simulink model "Duocopter_APID_Model"  (R2024b)
settings: Solver=VariableStepAuto  StartTime=0.0  StopTime=10.0  RelTol=1e-3
undefined symbols (not defined in the file): DiscIntNeverNeededParam, Discrete, Time
libraries: ctrlSharedLib x1, slpidlib x1
settings Model: Creator=charlemagne  LastModifiedBy=Nicol

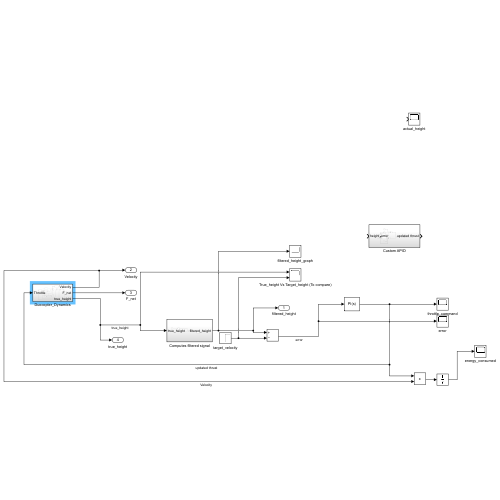
[thumbnail: Simulink's stored preview of the top-level diagram]
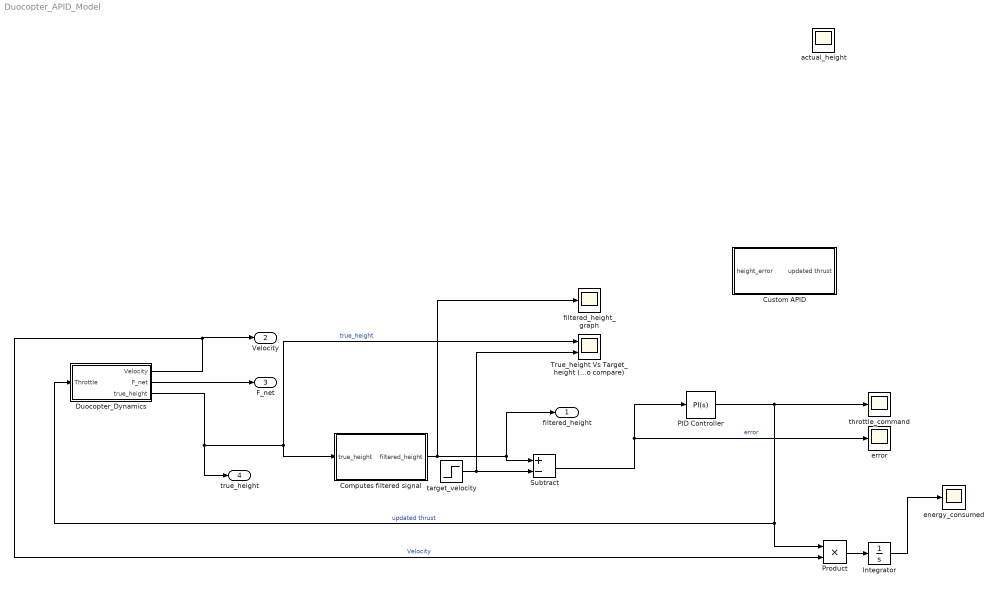
== system Duocopter_APID_Model ==
  Computes filtered signal : Subsystem
  Custom APID : Subsystem
  Duocopter_Dynamics : Subsystem
  Integrator : Integrator
  PID Controller : slpidlib/PID Controller  Controller=PI  Form=Parallel  TimeDomain=Continuous-time  UseExternalTs=off  SampleTime=-1  IntegratorMethod=Forward Euler  FilterMethod=Forward Euler  ControllerParametersSource=internal  P=120  I=80  UseKiTs=off  D=0  UseExternalDerivativeSource=off  N=100  UseFilter=on  TunerSelectOption=Transfer Function Based (PID Tuner App)  InitialConditionSource=internal  InitialConditionForIntegrator=0  InitialConditionForFilter=0  DifferentiatorICPrevScaledInput=0  ExternalReset=none  TrackingMode=off  Kt=1  LimitOutput=off  SatLimitsSource=internal  UpperSaturationLimit=inf  LowerSaturationLimit=-inf  LinearizeAsGain=on  AntiWindupMode=none  Kb=1  LimitIntegrator=off  UpperIntegratorSaturationLimit=inf  LowerIntegratorSaturationLimit=-inf  POutMin=[]  POutMax=[]  IOutMin=[]  IOutMax=[]  DOutMin=[]  DOutMax=[]  NOutMin=[]  NOutMax=[]  SumOutMin=[]  SumOutMax=[]  SaturationOutMin=[]  SaturationOutMax=[]  PParamMin=[]  PParamMax=[]  IParamMin=[]  IParamMax=[]  DParamMin=[]  DParamMax=[]  NParamMin=[]  NParamMax=[]  KbParamMin=[]  KbParamMax=[]  KtParamMin=[]  KtParamMax=[]  KbOutMin=[]  KbOutMax=[]  KtOutMin=[]  KtOutMax=[]  IntegratorOutMin=[]  IntegratorOutMax=[]  FilterOutMin=[]  FilterOutMax=[]  SumI1OutMin=[]  SumI1OutMax=[]  SumI2OutMin=[]  SumI2OutMax=[]  SumI3OutMin=[]  SumI3OutMax=[]  SumI4OutMin=[]  SumI4OutMax=[]  SumDOutMin=[]  SumDOutMax=[]  DifferentiatorOutMin=[]  DifferentiatorOutMax=[]  FilterDiffOutCoefMin=[]  FilterDiffOutCoefMax=[]  ReciprocalOutMin=[]  ReciprocalOutMax=[]  SumDenOutMin=[]  SumDenOutMax=[]  SumNumOutMin=[]  SumNumOutMax=[]  DivideOutMin=[]  DivideOutMax=[]  UdiffTsProdOutMin=[]  UdiffTsProdOutMax=[]  NTsProdOutMin=[]  NTsProdOutMax=[]  UintegralTsProdOutMin=[]  UintegralTsProdOutMax=[]  UngainTsProdOutMin=[]  UngainTsProdOutMax=[]  ClampingZeroOutDataTypeStr=Inherit: Inherit via back propagation  ClampingZeroOutMin=[]  ClampingZeroOutMax=[]  FilterDenConstantOutDataTypeStr=Inherit: Inherit via back propagation  FilterDenConstantOutMin=[]  FilterDenConstantOutMax=[]  PCopyOutDataTypeStr=Inherit: Inherit via back propagation  PCopyOutMin=[]  PCopyOutMax=[]  NCopyOutDataTypeStr=Inherit: Inherit via back propagation  NCopyOutMin=[]  NCopyOutMax=[]  IntegratorContinuousStateAttributes=''  IntegratorStateMustResolveToSignalObject=off  IntegratorRTWStateStorageClass=Auto  FilterContinuousStateAttributes=''  FilterStateMustResolveToSignalObject=off  FilterRTWStateStorageClass=Auto  ParallelPVariant=InternalParameters  IdealPVariant=Disabled  IVariant=InternalParameters  DVariant=Disabled  IntegratorVariant=Continuous  SatVariant=Disabled  AWVariant=Passthrough  PCopyVariant=Disabled  TRVariant=Disabled  FdbkBlocksVariant=Forward  IdealPFdbkVariant=Disabled  SatFdbkVariant=Disabled  DerivativeFilterVariant=Disabled  NVariant=Disabled  NCopyVariant=Disabled_SignalSpec  FilterICVariant=Disabled  IntegratorICVariant=InternalICs  ExternalResetVariant=Disabled  TRSumVariant=Passthrough  SumFdbkVariant=Disabled  SumVariant=Sum_PI  TsampFilterVariant=InternalTs  TsampNgainVariant=Passthrough  TsampIntegralVariant=Disabled_SignalSpec  ExternalSaturationOutDataTypeStr=Inherit: Same as second input  DerivativeSourceVariant=Disabled  PreIntVariant=InternalPreInt
  Product : Product
  Subtract : Sum  Inputs=+-
  True_height Vs Target_height (To compare) : Scope  NumInputPorts=2
  actual_height : Scope
  energy_consumed : Scope
  error : Scope
  filtered_height_graph : Scope
  target_velocity : Step  SampleTime=0
  throttle_command : Scope
  filtered_height : Outport
  Velocity : Outport  Port=2
  F_net : Outport  Port=3
  true_height : Outport  Port=4
  wires:
  Computes filtered signal/1(filtered_height) -> filtered_height_graph/1, filtered_height/1, Subtract/1
  Duocopter_Dynamics/1(Velocity) -> Product/2, Velocity/1  "Velocity"
  Duocopter_Dynamics/2(F_net) -> F_net/1
  Duocopter_Dynamics/3(true_height) -> true_height/1, True_height Vs Target_height (To compare)/1, Computes filtered signal/1(true_height)  "true_height"
  Subtract/1 -> PID Controller/1, error/1  "error"
  PID Controller/1 -> Duocopter_Dynamics/1(Throttle), Product/1, throttle_command/1  "updated thrust"
  target_velocity/1 -> True_height Vs Target_height (To compare)/2, Subtract/2
  Product/1 -> Integrator/1
  Integrator/1 -> energy_consumed/1

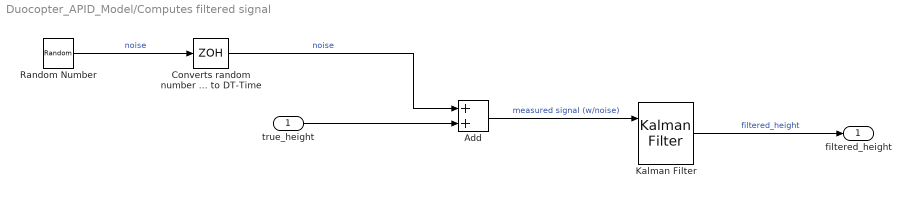
== system Duocopter_APID_Model/Computes filtered signal ==
  true_height : Inport
  Add : Sum
  Converts random number gen to DT-Time : ZeroOrderHold  SampleTime=-1
  Kalman Filter : ctrlSharedLib/Kalman Filter  TimeDomain=Discrete-Time  UseCurrentEstimator=on  ModelSource=LTI State-Space Variable  ModelSourceVariable=ss(0.95,1,1,0,1)  A=0.95  B=1  C=1  D=0  NumberOfStates=1  NumberOfInputs=1  NumberOfOutputs=1  InitialEstimateSource=Dialog  X0=0  P0=10  UseK=off  UseGH=off  NumberOfProcessNoiseInputs=1  G=1  TimeInvariantG=on  H=0  TimeInvariantH=on  Q=0.05  TimeInvariantQ=on  R=1  TimeInvariantR=on  N=0  TimeInvariantN=on  AddInputPort=on  AddEnablePort=off  OutputEstimatedY=off  OutputP=off  Ts=-1
  Random Number : RandomNumber  SampleTime=0.1
  filtered_height : Outport
  wires:
  Add/1 -> Kalman Filter/1  "measured signal (w/noise)"
  true_height/1 -> Add/2
  Kalman Filter/1 -> filtered_height/1  "filtered_height"
  Random Number/1 -> Converts random number gen to DT-Time/1  "noise"
  Converts random number gen to DT-Time/1 -> Add/1  "noise"

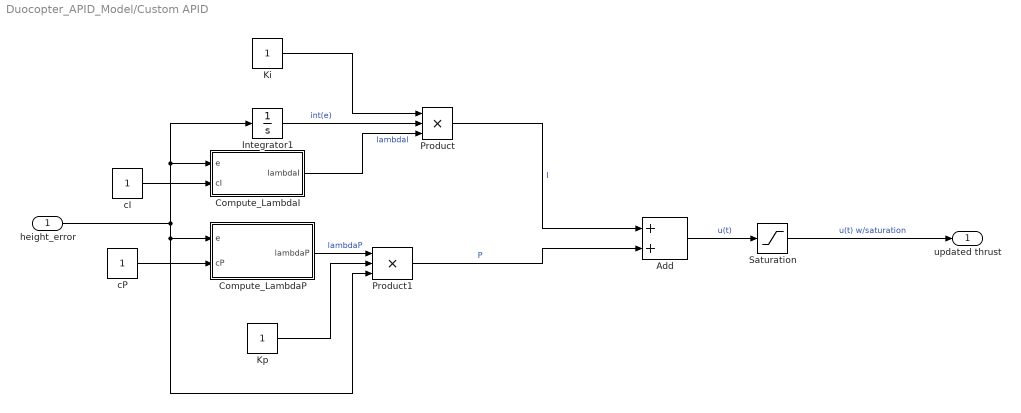
== system Duocopter_APID_Model/Custom APID ==
  height_error : Inport
  Add : Sum
  Compute_LambdaI : MATLAB Function  TreatAsAtomicUnit=on
  Compute_LambdaP : MATLAB Function  TreatAsAtomicUnit=on
  Integrator1 : Integrator
  Ki : Constant
  Kp : Constant
  Product : Product  Inputs=3
  Product1 : Product  Inputs=3
  Saturation : Saturate  UpperLimit=100  LowerLimit=0
  cI : Constant
  cP : Constant
  updated thrust : Outport
  wires:
  Product1/1 -> Add/2  "P"
  Compute_LambdaP/1(lambdaP) -> Product1/1  "lambdaP"
  Integrator1/1 -> Product/2  "int(e)"
  cI/1 -> Compute_LambdaI/2(cI)
  cP/1 -> Compute_LambdaP/2(cP)
  Kp/1 -> Product1/2
  Ki/1 -> Product/1
  Product/1 -> Add/1  "I"
  Saturation/1 -> updated thrust/1  "u(t) w/saturation"
  Add/1 -> Saturation/1  "u(t)"
  height_error/1 -> Product1/3, Compute_LambdaP/1(e), Integrator1/1, Compute_LambdaI/1(e)
  Compute_LambdaI/1(lambdaI) -> Product/3  "lambdal"

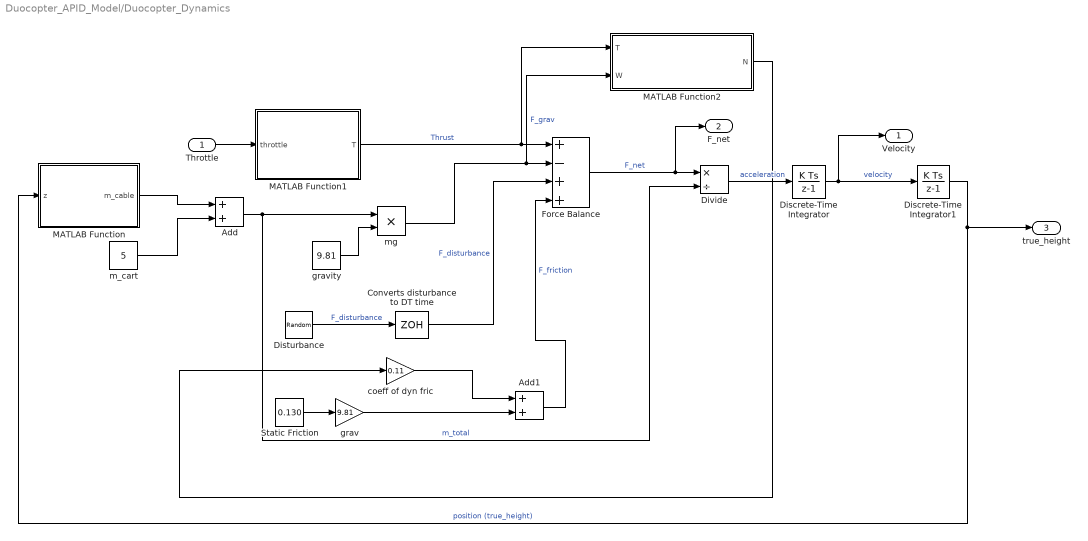
== system Duocopter_APID_Model/Duocopter_Dynamics ==
  Throttle : Inport
  Add : Sum
  Add1 : Sum
  Converts disturbance to DT time : ZeroOrderHold  SampleTime=0.01
  Discrete-Time Integrator : DiscreteIntegrator  SampleTime=-1  ICPrevOutput=DiscIntNeverNeededParam  ICPrevScaledInput=DiscIntNeverNeededParam
  Discrete-Time Integrator1 : DiscreteIntegrator  SampleTime=-1  ICPrevOutput=DiscIntNeverNeededParam  ICPrevScaledInput=DiscIntNeverNeededParam
  Disturbance : RandomNumber  SampleTime=0.1
  Divide : Product  Inputs=*/
  Force Balance : Sum  Inputs=+-++
  MATLAB Function : MATLAB Function  TreatAsAtomicUnit=on
  MATLAB Function1 : MATLAB Function  TreatAsAtomicUnit=on
  MATLAB Function2 : MATLAB Function  TreatAsAtomicUnit=on
  Static Friction : Constant  Value=0.130
  coeff of dyn fric : Gain  Gain=0.11
  grav : Gain  Gain=9.81
  gravity : Constant  Value=9.81
  m_cart : Constant  Value=5
  mg : Product
  Velocity : Outport
  F_net : Outport  Port=2
  true_height : Outport  Port=3
  wires:
  Divide/1 -> Discrete-Time Integrator/1  "acceleration"
  Throttle/1 -> MATLAB Function1/1(throttle)
  gravity/1 -> mg/2
  Force Balance/1 -> F_net/1, Divide/1  "F_net"
  coeff of dyn fric/1 -> Add1/1
  Discrete-Time Integrator/1 -> Velocity/1, Discrete-Time Integrator1/1  "velocity"
  Add/1 -> Divide/2, mg/1  "m_total"
  Discrete-Time Integrator1/1 -> MATLAB Function/1(z), true_height/1  "position (true_height)"
  mg/1 -> MATLAB Function2/2(W), Force Balance/2  "F_grav"
  Disturbance/1 -> Converts disturbance to DT time/1  "F_disturbance"
  m_cart/1 -> Add/2
  MATLAB Function/1(m_cable) -> Add/1
  MATLAB Function2/1(N) -> coeff of dyn fric/1
  MATLAB Function1/1(T) -> MATLAB Function2/1(T), Force Balance/1  "Thrust"
  Converts disturbance to DT time/1 -> Force Balance/3  "F_disturbance"
  Static Friction/1 -> grav/1
  grav/1 -> Add1/2
  Add1/1 -> Force Balance/4  "F_friction"

== matlab function Duocopter_APID_Model/Duocopter_Dynamics/MATLAB Function ==
  data: z input; m_cable output
function m_cable = piecewise_cable(z)
    % Define piecewise thresholds and masses
    z1 = 0.2;      % height at which cable starts lifting
    z2 = 0.6;      % height at which cable is fully extended
    m0 = 0.01;     % base cable mass (slack)
    m1 = 0.06;     % full cable mass when fully extended

    % Piecewise logic
    if z <= z1
        m_cable = m0;
    elseif z <= z2
        m_cable = m0 + ((m1 - m0) * (z - z1) / (z2 - z1));
    else
        m_cable = m1;
    end
end

== matlab function Duocopter_APID_Model/Custom APID/Compute_LambdaI ==
  data: e input; lambdaI output; cI input
function lambdaI = lambda_I_tanh(e, cI)
%e is the control error
%cI is the scaling factor for I gain
    lambdaI = tanh(cI * e);
end

== matlab function Duocopter_APID_Model/Custom APID/Compute_LambdaP ==
  data: e input; lambdaP output; cP input
function lambdaP = lambda_P_tanh(e, cP)
%e is the control error
%cP  is the scaling factor for P gain
    lambdaP = tanh(cP * e);
end

== matlab function Duocopter_APID_Model/Duocopter_Dynamics/MATLAB Function2 ==
  data: T input; N output; W input
function N = computeNormalForce(T, W)

%   T - Thrust [N]
%   W - Weight [N]


    x_thrust = 0.0115;  % [m]
    x_arm = 0.0065;     % [m]
    z_pad = 0.17;       % [m]

    N = (x_thrust * T - x_arm * W) / z_pad;
end

== matlab function Duocopter_APID_Model/Duocopter_Dynamics/MATLAB Function1 ==
  data: throttle input; T output
function T = throttle_to_thrust(throttle)
    % Constants
    T_max = 12.0; % Maximum thrust in Newtons at 100% throttle

    % Scale throttle (0–100) linearly to thrust
    T = (throttle / 100) * T_max;
end
